simulink model "fopiiTuningDiscrete"  (R2022b)
settings: Solver=FixedStepAuto  StartTime=0.0  StopTime=300  FixedStep=1  RelTol=1e-3
undefined symbols (not defined in the file or in its folder): DiscIntNeverNeededParam, kp, ti1, ti2
libraries: cstblocks x5, simulink x1
settings Model: Creator=jairo  LastModifiedBy=jairo
settings DataIOCC: ReturnWorkspaceOutputs=off

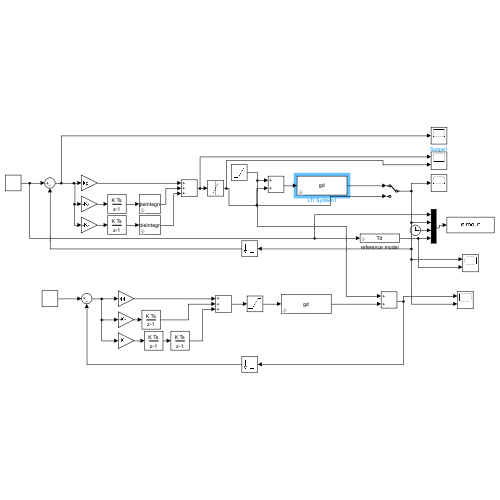
[thumbnail: Simulink's stored preview of the top-level diagram]
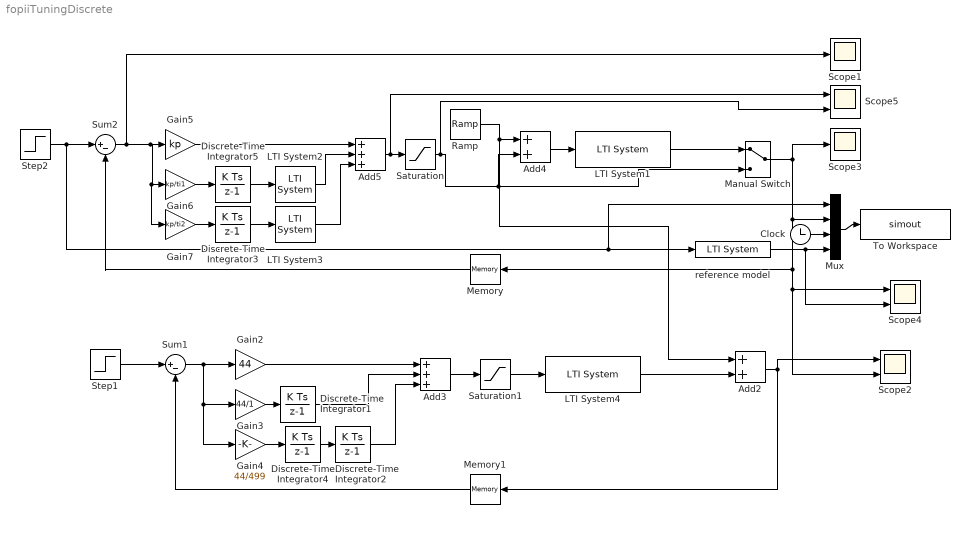
== system fopiiTuningDiscrete ==
  Add2 : Sum
  Add3 : Sum  Inputs=+++
  Add4 : Sum
  Add5 : Sum  Inputs=+++
  Clock : Clock
  Discrete-Time Integrator{1..5} (5 alike) : DiscreteIntegrator  SampleTime=-1  ICPrevOutput=DiscIntNeverNeededParam  ICPrevScaledInput=DiscIntNeverNeededParam
  Gain2 : Gain  Gain=44
  Gain3 : Gain  Gain=44/1
  Gain4 : Gain  Gain=44/499
  Gain5 : Gain  Gain=kp
  Gain6 : Gain  Gain=kp/ti1
  Gain7 : Gain  Gain=kp/ti2
  LTI System1 : cstblocks/LTI System  sys=gd  IC=[]
  LTI System2 : cstblocks/LTI System  sys=singleIntegrator  IC=[]
  LTI System3 : cstblocks/LTI System  sys=doubleIntegrator  IC=[]
  LTI System4 : cstblocks/LTI System  sys=gd  IC=[]
  Manual Switch : ManualSwitch
  Memory : Memory
  Memory1 : Memory
  Mux : Mux
  Ramp : simulink/Sources/Ramp  slope=-0.5  start=0  InitialOutput=0
  Saturation : Saturate  UpperLimit=255  LowerLimit=-255
  Saturation1 : Saturate  UpperLimit=255  LowerLimit=-255
  Scope1 : Scope
  Scope2 : Scope  NumInputPorts=2
  Scope3 : Scope
  Scope4 : Scope  NumInputPorts=2
  Scope5 : Scope  NumInputPorts=2
  Step1 : Step  Time=0  SampleTime=0
  Step2 : Step  Time=0  SampleTime=0
  Sum1 : Sum  Inputs=|+-
  Sum2 : Sum  Inputs=|+-
  To Workspace : ToWorkspace  VariableName=simout  SampleTime=-1
  reference model : cstblocks/LTI System  sys=Td  IC=[]
  wires:
  Discrete-Time Integrator3/1 -> LTI System3/1
  Gain5/1 -> Add5/1
  LTI System2/1 -> Add5/2
  Sum2/1 -> Scope1/1, Gain7/1, Gain6/1, Gain5/1
  Step2/1 -> Mux/1, reference model/1, Sum2/1
  Gain7/1 -> Discrete-Time Integrator3/1
  Add5/1 -> Scope5/1, Saturation/1
  LTI System3/1 -> Add5/3
  Add4/1 -> LTI System1/1
  Saturation/1 -> Manual Switch/2, Add4/2, Scope5/2
  Mux/1 -> To Workspace/1
  Manual Switch/1 -> Scope3/1, Scope4/1, Scope2/2, Memory/1, Mux/2
  Clock/1 -> Mux/3
  Gain4/1 -> Discrete-Time Integrator4/1
  Discrete-Time Integrator1/1 -> Add3/2
  Add3/1 -> Saturation1/1
  Step1/1 -> Sum1/1
  Gain2/1 -> Add3/1
  Ramp/1 -> Add2/1, Add4/1
  Add2/1 -> Scope2/1, Memory1/1
  Discrete-Time Integrator2/1 -> Add3/3
  LTI System4/1 -> Add2/2
  Gain3/1 -> Discrete-Time Integrator1/1
  Discrete-Time Integrator4/1 -> Discrete-Time Integrator2/1
  Sum1/1 -> Gain4/1, Gain3/1, Gain2/1
  Gain6/1 -> Discrete-Time Integrator5/1
  reference model/1 -> Scope4/2, Mux/4
  Discrete-Time Integrator5/1 -> LTI System2/1
  Memory/1 -> Sum2/2
  Memory1/1 -> Sum1/2
  Saturation1/1 -> LTI System4/1
  LTI System1/1 -> Manual Switch/1
